simulink model "pid_1"  (Simulink 6.4)
settings: Solver=ode45  StartTime=0.0  StopTime=10.0  RelTol=1e-3
settings Model: LastModifiedBy=Administrator

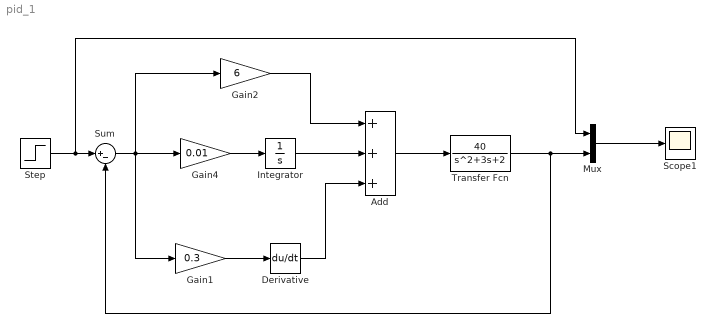
== system pid_1 ==
  Add : Sum  Inputs=+++  OutScaling=2^-10
  Derivative : Derivative
  Gain1 : Gain  Gain=0.3  SaturateOnIntegerOverflow=on
  Gain2 : Gain  Gain=6  SaturateOnIntegerOverflow=on
  Gain4 : Gain  Gain=0.01  SaturateOnIntegerOverflow=on
  Integrator : Integrator
  Mux : Mux  Inputs=2
  Scope1 : Scope
  Step : Step  SampleTime=0
  Sum : Sum  Inputs=|+-
  Transfer Fcn : TransferFcn  Numerator=[40]  Denominator="[1 3 2   ]"
  wires:
  Step/1 -> Sum/1, Mux/1
  Gain2/1 -> Add/1
  Gain1/1 -> Derivative/1
  Derivative/1 -> Add/3
  Add/1 -> Transfer Fcn/1
  Transfer Fcn/1 -> Mux/2, Sum/2
  Mux/1 -> Scope1/1
  Integrator/1 -> Add/2
  Gain4/1 -> Integrator/1
  Sum/1 -> Gain4/1, Gain2/1, Gain1/1
